simulink model "TRAS_azimuth_model"  (Simulink 9.1)
settings: Solver=ode5  StartTime=0.0  StopTime=30  FixedStep=.01  RelTol=1e-3  EnableMultiTasking=on
PreLoadFcn:
  | load tras_char
undefined symbols (not defined in the file): control_a, force_a, rpm_a
settings Model: Creator=inteco  LastModifiedBy=inteco
settings DataIOCC: LimitDataPoints=on  SignalLoggingSaveFormat=ModelDataLogs  SignalLoggingName=sigsOut
settings OptimizationCC: ExpressionDepthLimit=2147483647
settings DebuggingCC: SaveWithParameterizedLinksMsg=none  SignalResolutionControl=TryResolveAllWithWarning  MultiTaskDSMMsg=warning  MultiTaskCondExecSysMsg=none  FcnCallInpInsideContextMsg=warning  StateNameClashWarn=warning
settings HardwareCC: TargetUnknown=on
settings GRTTargetCC: GeneratePreprocessorConditionals=Disable all
settings ConfigComp: CovSFcnEnable=off

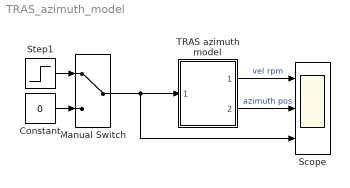
== system TRAS_azimuth_model ==
  Constant : Constant  Value=0
  Manual Switch : ManualSwitch
  Scope : Scope  NumInputPorts=3
  Step1 : Step  After=.2  SampleTime=0
  TRAS azimuth model : Subsystem
  wires:
  TRAS azimuth model/1(rpm_a) -> Scope/1  "vel rpm"
  TRAS azimuth model/2(pos_am) -> Scope/2  "azimuth pos"
  Manual Switch/1 -> TRAS azimuth model/1("ctrl_a "), Scope/3
  Step1/1 -> Manual Switch/1
  Constant/1 -> Manual Switch/2

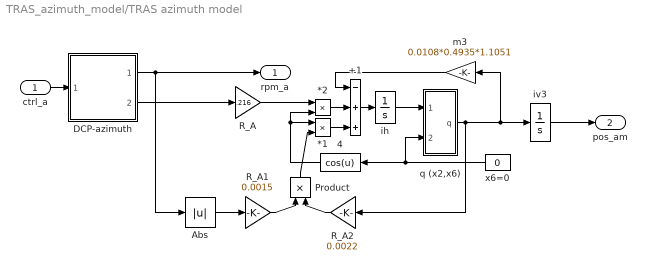
== system TRAS_azimuth_model/TRAS azimuth model ==
  "ctrl_a " : Inport
  *1 : Product  SaturateOnIntegerOverflow=on  InputSameDT=on  OutDataTypeStr=Inherit: Same as first input
  *2 : Product  SaturateOnIntegerOverflow=on  InputSameDT=on  OutDataTypeStr=Inherit: Same as first input
  +1 : Sum  Inputs=-++  SaturateOnIntegerOverflow=on  InputSameDT=on  OutDataTypeStr=Inherit: Same as first input
  4 : Fcn  Expr=cos(u)
  Abs : Abs  SaturateOnIntegerOverflow=on
  DCP-azimuth : Subsystem
  Product : Product  SaturateOnIntegerOverflow=on  InputSameDT=on  OutDataTypeStr=Inherit: Same as first input
  R_A : Gain  Gain=.216  OutDataTypeStr=Inherit: Same as input  ParamDataTypeStr=Inherit: Same as input
  R_A1 : Gain  Gain=0.0015  OutDataTypeStr=Inherit: Same as input  ParamDataTypeStr=Inherit: Same as input
  R_A2 : Gain  Gain=0.0022  OutDataTypeStr=Inherit: Same as input  ParamDataTypeStr=Inherit: Same as input
  ih : Integrator
  iv3 : Integrator
  m3 : Gain  Gain=0.0108*0.4935*1.1051  OutDataTypeStr=Inherit: Same as input  ParamDataTypeStr=Inherit: Same as input
  q (x2,x6) : Subsystem
  x6=0 : Constant  Value=0
  rpm_a : Outport
  pos_am : Outport  Port=2
  wires:
  DCP-azimuth/2(FORCE_A) -> R_A/1
  *1/1 -> +1/3
  m3/1 -> +1/1
  4/1 -> *1/1, *2/2
  *2/1 -> +1/2
  ih/1 -> q (x2,x6)/1(x2)
  q (x2,x6)/1(q) -> iv3/1, m3/1, R_A2/1
  R_A/1 -> *2/1
  +1/1 -> ih/1
  x6=0/1 -> q (x2,x6)/2(x6), 4/1
  "ctrl_a "/1 -> DCP-azimuth/1(CTR_A)
  iv3/1 -> pos_am/1
  DCP-azimuth/1(RPM_A) -> rpm_a/1, Abs/1
  Product/1 -> *1/2
  R_A2/1 -> Product/2
  R_A1/1 -> Product/1
  Abs/1 -> R_A1/1

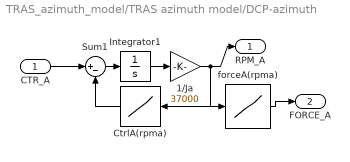
== system TRAS_azimuth_model/TRAS azimuth model/DCP-azimuth ==
  CTR_A : Inport
  1/Ja : Gain  Gain=37000  SaturateOnIntegerOverflow=on  OutDataTypeStr=Inherit: Same as input  ParamDataTypeStr=Inherit: Same as input
  CtrlA(rpma) : Lookup  InputValues=rpm_a  Table=control_a  SaturateOnIntegerOverflow=on
  Integrator1 : Integrator
  Sum1 : Sum  Inputs=|+-  SaturateOnIntegerOverflow=on  InputSameDT=on  OutDataTypeStr=Inherit: Same as first input
  forceA(rpma) : Lookup  InputValues=rpm_a  Table=force_a  SaturateOnIntegerOverflow=on
  RPM_A : Outport
  FORCE_A : Outport  Port=2
  wires:
  Sum1/1 -> Integrator1/1
  CtrlA(rpma)/1 -> Sum1/2
  Integrator1/1 -> 1/Ja/1
  1/Ja/1 -> CtrlA(rpma)/1, forceA(rpma)/1, RPM_A/1
  CTR_A/1 -> Sum1/1
  forceA(rpma)/1 -> FORCE_A/1

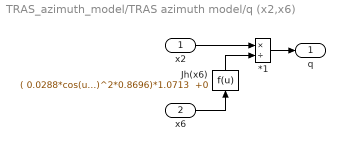
== system TRAS_azimuth_model/TRAS azimuth model/q (x2,x6) ==
  x2 : Inport
  x6 : Inport  Port=2
  " Jh(x6)" : Fcn  Expr="( 0.0288*cos(u)^2*0.8696)*1.0713  +0"
  *1 : Product  Inputs=*/  SaturateOnIntegerOverflow=on  InputSameDT=on  OutDataTypeStr=Inherit: Same as first input
  q : Outport
  wires:
  *1/1 -> q/1
  x2/1 -> *1/1
  x6/1 -> " Jh(x6)"/1
  " Jh(x6)"/1 -> *1/2
